simulink model "DSPequivalent_FOC_2020a"  (R2020a)
settings: Solver=ode5  StartTime=0.0  StopTime=tend  FixedStep=Tsim  RelTol=1e-3
values from neighbouring files (symbols this model uses):
  alpha = 0.091    [init_DSPeq_FOC.m]    (also in init_DSPeq_IM.m = 0.04; paramSet.m = 0.04)
  d = 0.444    [FRAexport_2.m]    (also in init_DSPeq_FOC.m = 0.78975)
  DEADTIME = 100    [init_DSPeq_FOC.m]    (also in init_DSPeq_IM.m)
  emf = psi*we    [init_DSPeq_FOC.m]
  f_ref = 270    [init_DSPeq_FOC.m]    (also in init_DSPeq_IM.m = 50)
  Id_ref = 0    [init_DSPeq_FOC.m]    (also in init_DSPeq_IM.m = 1; step_prikaz.m = Idq2(:,2))
  Iq_ref = 2    [init_DSPeq_FOC.m]    (also in init_DSPeq_IM.m = 1; step_prikaz.m = Idq2(:,3))
  ISENSE_SCALE = 10    [init_DSPeq_FOC.m]    (also in init_DSPeq_IM.m)
  Ki = 0.2/ur    (= 0.05)    [init_DSPeq.m]    (also in init_DSPeq_FOC.m = wc*Kp/(tan(-pi/2+pm+2*atan(wc*Ts/4)+atan(wc*L/R))))
  Kp = 1.8    [init_DSPeq.m]    (also in init_DSPeq_FOC.m = R*sqrt(1+(wc*L/R)^2))
  L = 3.4e-3    (= 0.0034)    [init_DSPeq_FOC.m]
  Nos = 16    [init_DSPeq.m]    (also in init_DSPeq_FOC.m; init_DSPeq_IM.m)
  ofst_a = 0    [init_DSPeq_FOC.m]
  ofst_b = 0    [init_DSPeq_FOC.m]
  OVERSAMPLING = 1    [init_DSPeq.m]    (also in init_DSPeq_FOC.m; init_DSPeq_IM.m; raw_plot.m)
  p = 3    [init_DSPeq_FOC.m]    (also in init_DSPeq_IM.m = 1)
  ph = pi    (= 3.14159265359)    [init_DSPeq_FOC.m]
  PWM_TBPRD = 4992    [init_DSPeq.m]    (also in init_DSPeq_FOC.m; init_DSPeq_IM.m; paramSet.m)
  R = 9.92e3    (= 9920)    [init_DSPeq.m]    (also in init_DSPeq_FOC.m = 0.47)
  Tadc_exe = Tadc    (= 6.24e-06)    [init_DSPeq_FOC.m]
  tau_fil = 5e-6    (= 5e-06)    [init_DSPeq_FOC.m]
  tfra = 0.33    [init_DSPeq_FOC.m]
  Tpwm = 2*PWM_TBPRD/ftbclk    (= 9.984e-05)    [init_DSPeq.m]    (also in init_DSPeq_FOC.m; init_DSPeq_IM.m; paramSet.m)
  tref = dmacnt_ref*Ts    [init_DSPeq_FOC.m]
  Ts = Tpwm/ur    (= 2.496e-05)    [init_DSPeq.m]    (also in init_DSPeq_FOC.m = 4.992e-05; init_DSPeq_IM.m = 4.992e-05; paramSet.m = 4.992e-05; step_prikaz.m = Ts/1000)
  Ts_cmp = Ts    (= 4.992e-05)    [init_DSPeq_FOC.m]
  Ts_exe = Ts    (= 4.992e-05)    [init_DSPeq_FOC.m]
  Ttbclk = 1/ftbclk    (= 1e-08)    [init_DSPeq.m]    (also in init_DSPeq_FOC.m; init_DSPeq_IM.m; paramSet.m)
  Udol = 0    [init_DSPeq_FOC.m]    (also in init_DSPeq_IM.m = UD_MAX/2)
  Udq0 = [0; 0]    [init_DSPeq_FOC.m]
  Udq_max = E/2    (= 260)    [init_DSPeq_FOC.m]    (also in init_DSPeq_IM.m = E/(2*sqrt(2)))
  Uqol = 0    [init_DSPeq_FOC.m]    (also in init_DSPeq_IM.m)
  ur = 4    [init_DSPeq.m]    (also in init_DSPeq_FOC.m = 2; init_DSPeq_IM.m = 2; paramSet.m = 2; raw_plot.m = 2)
  we = 2*pi*f_ref    (= 1696.46003294)    [init_DSPeq_FOC.m]
  wm = we/p    (= 565.486677646)    [init_DSPeq_FOC.m]
undefined symbols (not defined in the file or in its folder): j, Ld, Lq
libraries: simulink x12, powerlib x5, slctrlblks x1
settings Model: Creator=ruzic  LastModifiedBy=ruzic
settings DataIOCC: ReturnWorkspaceOutputs=off
settings DebuggingCC: UnderSpecifiedDataTypeMsg=warning  UnderSpecifiedDimensionMsg=warning  ArithmeticOperatorsInVariantConditions=warning
settings SFSimCC: CustomCodeUndefinedFunction=UseInterfaceOnly

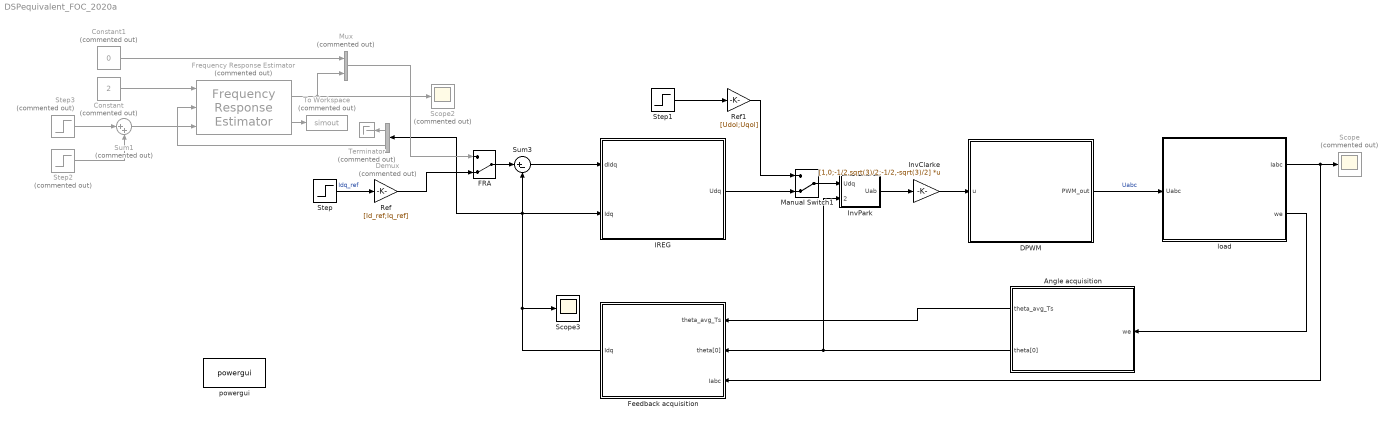
== system DSPequivalent_FOC_2020a ==
  Angle acquisition : Subsystem
  Constant : Constant  Commented=on  Value=2  SampleTime=Ts
  Constant1 : Constant  Commented=on  Value=0  SampleTime=Ts
  DPWM : Subsystem
  Demux : Demux  Commented=on  Outputs=2
  FRA : ManualSwitch  CurrentSetting=0
  Feedback acquisition : Subsystem
  Frequency Response Estimator : slctrlblks/Frequency Response Estimator  Commented=on  DiscreteTs=Ts  OutputMode=control action + perturbation  BlockDataType=double  SineSource=Block parameters  Frequencies=f_test  FreqUnits=Hz  Amplitudes=0.1  NumOfFreq=3  ExperimentMode=Sinestream  NumOfSetPeriod=2  NumOfEstPeriod=4  NumOfSlowestPeriod=3  EstimationMode=Offline  UseBodePlot=on  BaselinePlant=W1  PlotRefreshFactor=100  BodePlotChoice=VariantNull  ExperimentChoice=VariantSSNoEst  OutputChoice=VariantCandD
      settings: SourceProductBaseCode=SD
  IREG : Subsystem
  InvClarke : Gain  Gain=[1,0;-1/2,sqrt(3)/2;-1/2,-sqrt(3)/2]  Multiplication=Matrix(K*u)
  InvPark : Subsystem
  Manual Switch1 : ManualSwitch  CurrentSetting=0
  Mux : Mux  Commented=on  Inputs=2
  Ref : Gain  Gain=[Id_ref;Iq_ref]
  Ref1 : Gain  Gain=[Udol;Uqol]
  Scope : Scope  Commented=on
  Scope2 : Scope  Commented=on
  Scope3 : Scope
  Step : Step  Time=tref  Before=4/2  SampleTime=Ts_exe
  Step1 : Step  Time=Tpwm/ur  Before=Udq0  After=Udq0  SampleTime=Ts_exe
  Step2 : Step  Commented=on  Time=tref + tfra  After=-1  SampleTime=Ts
  Step3 : Step  Commented=on  Time=tref  SampleTime=Ts
  Sum1 : Sum  Commented=on  Inputs=|++
  Sum3 : Sum  Inputs=|+-
  Terminator : Terminator  Commented=on
  To Workspace : ToWorkspace  Commented=on  VariableName=simout  SaveFormat=Timeseries  SampleTime=-1
  load : Subsystem
  powergui : powerlib/powergui  Priority=1  SimulationMode=Continuous  SampleTime=50e-6  frequency=60  Iterations=50  frequencyindice=0  Pbase=100e6  ErrMax=1e-4  UnitsV=kV  UnitsW=MW  buscounter=0  FunctionMessages=off  echomessages=off  EnableUseOfTLC=off  CurrentSourceSwitches=off  DisableSnubberDevices=off  DisableRonSwitches=off  DisableVfSwitches=off  DisplayEquations=off  AutomaticDiscreteSolvers=off  SolverType=Tustin/Backward Euler (TBE)  Interpol=off  ExternalGateDelay=off  methode=off  Ts=100  x0status=blocks  SPID=on  SwTol=0  HookPort=off  NonlinearTolerance=1e-4  nMaxIteration=100  ContinueOnMaxIteration=off  RestoreLinks=warning  ResistiveCurrentMeasurement=off  Frange=[0:2:500]  Ylog=off  Xlog=on  ShowGrid=off  save=off  variable=ZData  structure=0  ZoomFFT=off  StartTime=0.0  cycles=1  DisplayStyle=1  fundamental=60  FreqAxis=off  MaxFrequency=1000  frequencyindicesteady=1  RmsSteady=1  display=off
  wires:
  Sum3/1 -> IREG/1(dIdq)
  Step/1 -> Ref/1  "Idq_ref"
  DPWM/1(PWM_out) -> load/1(Uabc)  "Uabc"
  Ref1/1 -> Manual Switch1/1
  InvPark/1(Uab) -> InvClarke/1
  InvClarke/1 -> DPWM/1(u)
  Angle acquisition/2(theta[0]) -> InvPark/2(theta), Feedback acquisition/2(theta[0])
  Step1/1 -> Ref1/1
  Feedback acquisition/1("Idq ") -> Scope3/1, IREG/2(Idq), Demux/1, Sum3/2
  Angle acquisition/1(theta_avg_Ts) -> Feedback acquisition/1(theta_avg_Ts)
  IREG/1(Udq) -> Manual Switch1/2
  Manual Switch1/1 -> InvPark/1(Udq)
  load/2(we) -> Angle acquisition/1(we)
  load/1(Iabc) -> Feedback acquisition/3(Iabc), Scope/1
  Mux/1 -> FRA/1
  Frequency Response Estimator/1 -> Mux/2, Scope2/1
  Constant/1 -> Frequency Response Estimator/1
  Demux/2 -> Frequency Response Estimator/2
  Demux/1 -> Terminator/1
  Constant1/1 -> Mux/1
  Frequency Response Estimator/2 -> To Workspace/1
  Sum1/1 -> Frequency Response Estimator/3
  Step2/1 -> Sum1/2
  Step3/1 -> Sum1/1
  FRA/1 -> Sum3/1
  Ref/1 -> FRA/2

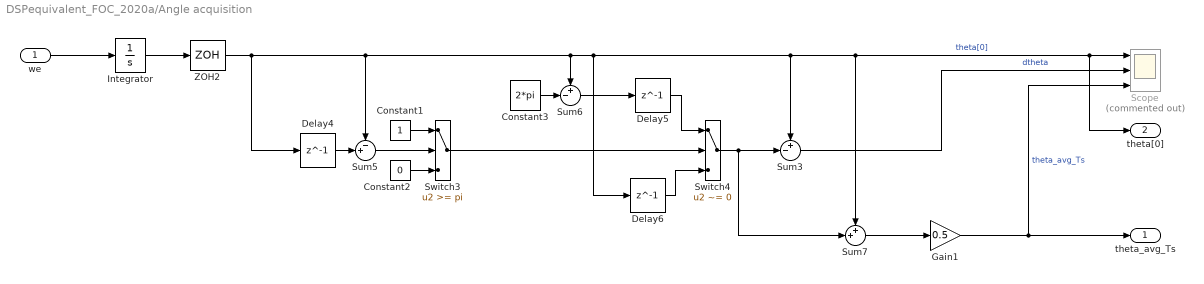
== system DSPequivalent_FOC_2020a/Angle acquisition ==
  we : Inport
  Constant1 : Constant
  Constant2 : Constant  Value=0
  Constant3 : Constant  Value=2*pi
  Delay4 : Delay  DelayLength=1
  Delay5 : Delay  DelayLength=1  SampleTime=Ts_exe
  Delay6 : Delay  DelayLength=1  SampleTime=Ts_exe
  Gain1 : Gain  Gain=0.5
  Integrator : Integrator  WrapState=on  WrappedStateUpperValue=2*pi  WrappedStateLowerValue=0
  Scope : Scope  Commented=on  NumInputPorts=3
  Sum3 : Sum  Inputs=+-|
  Sum5 : Sum  Inputs=-+|
  Sum6 : Sum  Inputs=+-|
  Sum7 : Sum  Inputs=++|
  Switch3 : Switch  Threshold=pi  OutDataTypeStr=boolean
  Switch4 : Switch  Criteria=u2 ~= 0
  ZOH2 : ZeroOrderHold  SampleTime=Ts_exe
  theta_avg_Ts : Outport  VectorParamsAs1DForOutWhenUnconnected=off
  theta[0] : Outport  Port=2  VectorParamsAs1DForOutWhenUnconnected=off
  wires:
  Integrator/1 -> ZOH2/1
  Sum3/1 -> Scope/2  "dtheta"
  Delay4/1 -> Sum5/2
  Sum5/1 -> Switch3/2
  Constant1/1 -> Switch3/1
  Constant2/1 -> Switch3/3
  Constant3/1 -> Sum6/2
  Switch3/1 -> Switch4/2
  Delay5/1 -> Switch4/1
  Switch4/1 -> Sum7/2, Sum3/2
  Delay6/1 -> Switch4/3
  Sum7/1 -> Gain1/1
  Sum6/1 -> Delay5/1
  we/1 -> Integrator/1
  ZOH2/1 -> Delay6/1, theta[0]/1, Scope/1, Sum7/1, Sum3/1, Sum6/1, Sum5/1, Delay4/1  "theta[0]"
  Gain1/1 -> theta_avg_Ts/1, Scope/3  "theta_avg_Ts"

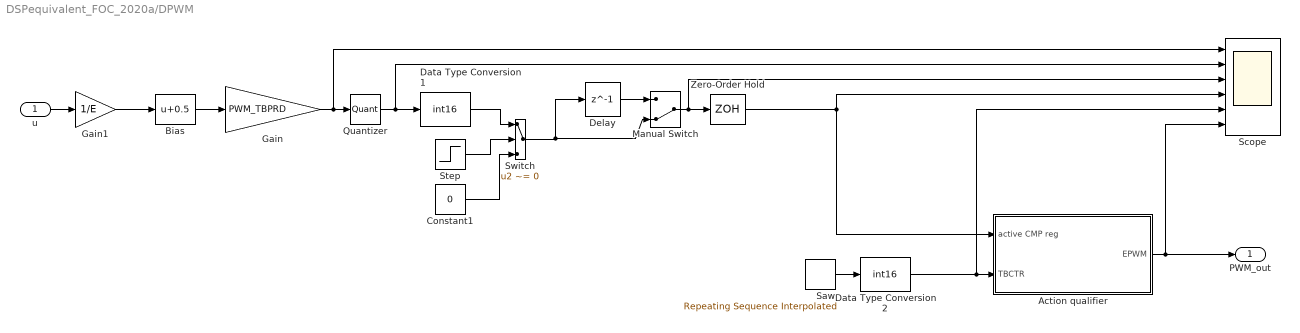
== system DSPequivalent_FOC_2020a/DPWM ==
  u : Inport
  Action qualifier : Subsystem
  Bias : Bias  Bias=0.5
  Constant1 : Constant  Value=0
  Data Type Conversion1 : DataTypeConversion  OutDataTypeStr=int16  ConvertRealWorld=Stored Integer (SI)  RndMeth=Round
  Data Type Conversion2 : DataTypeConversion  OutDataTypeStr=int16  ConvertRealWorld=Stored Integer (SI)  RndMeth=Round
  Delay : Delay  DelayLength=1  InitialCondition=0  SampleTime=Ts_exe
  Gain : Gain  Gain=PWM_TBPRD
  Gain1 : Gain  Gain=1/E
  Manual Switch : ManualSwitch  CurrentSetting=0
  Quantizer : Quantizer  QuantizationInterval=1
  Saw : simulink/Sources/Repeating Sequence Interpolated  OutValues=[0 PWM_TBPRD 1].'  TimeValues=[0 Tpwm/2 (Tpwm-Ttbclk)].'  LookUpMeth=Interpolation-Use End Values  tsamp=Ttbclk  OutMin=[]  OutMax=[]  OutDataTypeStr=double  OutputDataTypeScalingMode=double  OutDataType=fixdt(0,8)  OutScaling=2^-10
  Scope : Scope  NumInputPorts=6
  Step : Step  Time=Tpwm/ur
  Switch : Switch  Criteria=u2 ~= 0
  Zero-Order Hold : ZeroOrderHold  SampleTime=Ts_cmp
  PWM_out : Outport  VectorParamsAs1DForOutWhenUnconnected=off
  wires:
  u/1 -> Gain1/1
  Quantizer/1 -> Data Type Conversion1/1, Scope/2
  Saw/1 -> Data Type Conversion2/1
  Zero-Order Hold/1 -> Action qualifier/1(active CMP reg), Scope/4
  Action qualifier/1(EPWM) -> Scope/6, PWM_out/1
  Data Type Conversion1/1 -> Switch/1
  Data Type Conversion2/1 -> Scope/5, Action qualifier/2(TBCTR)
  Gain1/1 -> Bias/1
  Gain/1 -> Quantizer/1, Scope/1
  Bias/1 -> Gain/1
  Constant1/1 -> Switch/3
  Step/1 -> Switch/2
  Switch/1 -> Manual Switch/2, Delay/1
  Manual Switch/1 -> Scope/3, Zero-Order Hold/1
  Delay/1 -> Manual Switch/1

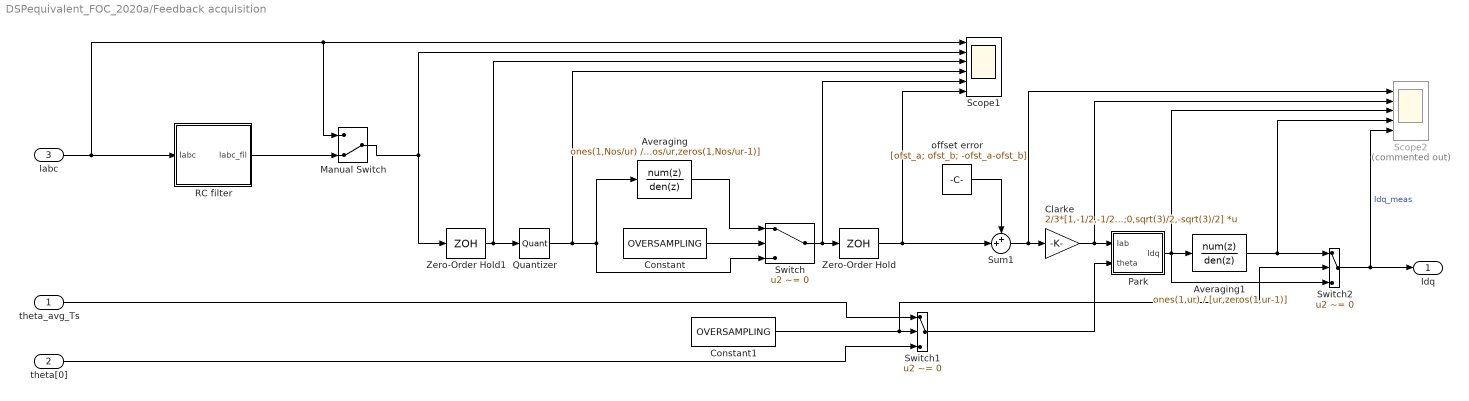
== system DSPequivalent_FOC_2020a/Feedback acquisition ==
  theta_avg_Ts : Inport
  theta[0] : Inport  Port=2
  Iabc : Inport  Port=3
  Averaging : DiscreteTransferFcn  Numerator=ones(1,Nos/ur)  Denominator=[Nos/ur,zeros(1,Nos/ur-1)]
  Averaging1 : DiscreteTransferFcn  Numerator=ones(1,ur)  Denominator=[ur,zeros(1,ur-1)]
  Clarke : Gain  Gain=2/3*[1,-1/2,-1/2;0,sqrt(3)/2,-sqrt(3)/2]  Multiplication=Matrix(K*u)
  Constant : Constant  Value=OVERSAMPLING
  Constant1 : Constant  Value=OVERSAMPLING
  Manual Switch : ManualSwitch  CurrentSetting=0
  Park : Subsystem
  Quantizer : Quantizer  QuantizationInterval=3/(2^12-1)*ISENSE_SCALE
  RC filter : Subsystem
  Scope1 : Scope  NumInputPorts=6
  Scope2 : Scope  Commented=on  NumInputPorts=5
  Sum1 : Sum  Inputs=++|
  Switch : Switch  Criteria=u2 ~= 0
  Switch1 : Switch  Criteria=u2 ~= 0
  Switch2 : Switch  Criteria=u2 ~= 0
  Zero-Order Hold : ZeroOrderHold  SampleTime=Ts_exe
  Zero-Order Hold1 : ZeroOrderHold  SampleTime=Tadc_exe
  offset error : Constant  Value=[ofst_a; ofst_b; -ofst_a-ofst_b]  SampleTime=Ts_exe
  "Idq " : Outport  VectorParamsAs1DForOutWhenUnconnected=off
  wires:
  Switch/1 -> Scope1/5, Zero-Order Hold/1
  Zero-Order Hold1/1 -> Scope1/3, Quantizer/1
  Quantizer/1 -> Scope1/4, Switch/3, Averaging/1
  Averaging/1 -> Switch/1
  Constant/1 -> Switch/2
  Constant1/1 -> Switch2/2, Switch1/2
  Switch2/1 -> Scope2/5, "Idq "/1  "Idq_meas"
  theta[0]/1 -> Switch1/3
  theta_avg_Ts/1 -> Switch1/1
  Averaging1/1 -> Scope2/4, Switch2/1
  Switch1/1 -> Park/2(theta)
  Clarke/1 -> Scope2/2, Park/1(Iab)
  Park/1(Idq) -> Switch2/3, Scope2/3, Averaging1/1
  Sum1/1 -> Scope2/1, Clarke/1
  Manual Switch/1 -> Scope1/2, Zero-Order Hold1/1
  Iabc/1 -> RC filter/1(Iabc), Manual Switch/1, Scope1/1
  RC filter/1(Iabc_fil) -> Manual Switch/2
  Zero-Order Hold/1 -> Scope1/6, Sum1/2
  offset error/1 -> Sum1/1

== system DSPequivalent_FOC_2020a/IREG ==
  dIdq : Inport
  Idq : Inport  Port=2
  Dif.comp. : Subsystem
  IMC : Subsystem
  Manual Switch : ManualSwitch
  Manual Switch1 : ManualSwitch
  PI error decoupl. : Subsystem
  PI feedback decoupl. : Subsystem
  Scope : Scope
  Udq : Outport  VectorParamsAs1DForOutWhenUnconnected=off
  wires:
  Manual Switch/1 -> Scope/1, Udq/1
  dIdq/1 -> PI feedback decoupl./1(dIdq), PI error decoupl./1(dIdq), IMC/1(dIdq)
  IMC/1(Out) -> Dif.comp./1(In)
  Dif.comp./1(Out) -> Manual Switch/1
  Idq/1 -> PI feedback decoupl./2(Idq)
  PI error decoupl./1(Out) -> Manual Switch1/1
  PI feedback decoupl./1(Out) -> Manual Switch1/2
  Manual Switch1/1 -> Manual Switch/2

== system DSPequivalent_FOC_2020a/InvPark ==
  Udq : Inport
  theta : Inport  Port=2
  Complex to Real-Imag1 : ComplexToRealImag
  Demux : Demux  Outputs=2
  Gain8 : Gain  Gain=1j
  Math Function1 : Math  SignedPower=on  OutputSignalType=complex  SaturateOnIntegerOverflow=on
  Mux3 : Mux  Inputs=2
  Product4 : Product
  Real-Imag to Complex1 : RealImagToComplex
  Uab : Outport  VectorParamsAs1DForOutWhenUnconnected=off
  wires:
  Real-Imag to Complex1/1 -> Product4/2
  Math Function1/1 -> Product4/1
  Complex to Real-Imag1/1 -> Mux3/1
  Gain8/1 -> Math Function1/1
  Demux/1 -> Real-Imag to Complex1/1  "ud"
  Mux3/1 -> Uab/1  "Uab"
  Product4/1 -> Complex to Real-Imag1/1
  Complex to Real-Imag1/2 -> Mux3/2
  Demux/2 -> Real-Imag to Complex1/2  "uq"
  theta/1 -> Gain8/1
  Udq/1 -> Demux/1

== system DSPequivalent_FOC_2020a/load ==
  Uabc : Inport
  Demux : Demux  Outputs=2
  Manual Switch : ManualSwitch  CurrentSetting=0
  Mux : Mux  Commented=on  Inputs=2
  Mux1 : Mux  Inputs=2
  PMSM : Subsystem
  RL + emf : Subsystem  Commented=on
  Iabc : Outport  VectorParamsAs1DForOutWhenUnconnected=off
  we : Outport  Port=2  VectorParamsAs1DForOutWhenUnconnected=off
  tag scope: iabc=global
  wires:
  Uabc/1 -> PMSM/1(Uabc), RL + emf/1(Uabc)
  Demux/1 -> [iabc], Iabc/1
  Mux/1 -> Manual Switch/1
  RL + emf/1(Iabc) -> Mux/1
  RL + emf/2(we) -> Mux/2
  Manual Switch/1 -> Demux/1
  Demux/2 -> we/1
  PMSM/1(Iabc) -> Mux1/1
  PMSM/2(we) -> Mux1/2
  Mux1/1 -> Manual Switch/2

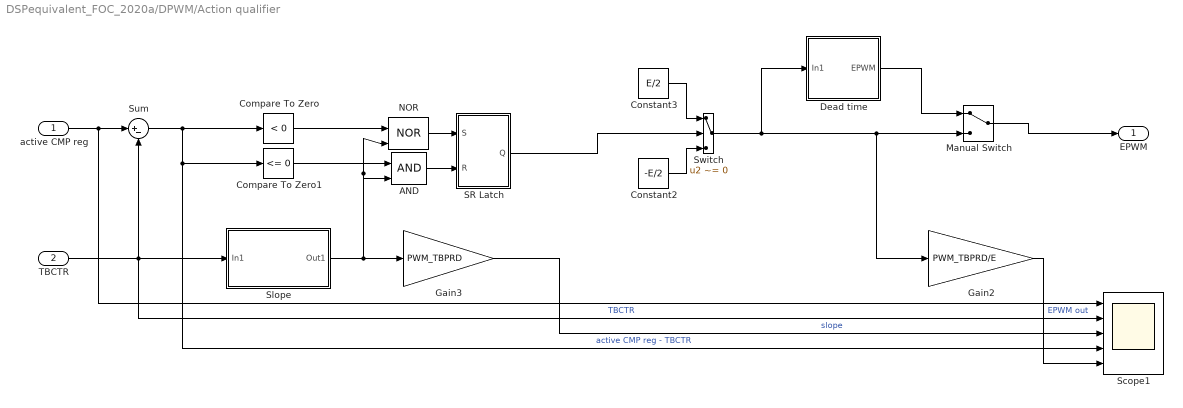
== system DSPequivalent_FOC_2020a/DPWM/Action qualifier ==
  active CMP reg : Inport
  TBCTR : Inport  Port=2
  AND : Logic  IconShape=distinctive  AllPortsSameDT=off  OutDataTypeStr=boolean
  Compare To Zero : simulink/Logic and Bit Operations/Compare To Zero  relop=<  OutDataTypeStr=boolean
  Compare To Zero1 : simulink/Logic and Bit Operations/Compare To Zero  relop=<=  OutDataTypeStr=boolean
  Constant2 : Constant  Value=-E/2
  Constant3 : Constant  Value=E/2
  Dead time : Subsystem
  Gain2 : Gain  Gain=PWM_TBPRD/E
  Gain3 : Gain  Gain=PWM_TBPRD
  Manual Switch : ManualSwitch
  NOR : Logic  Operator=NOR  IconShape=distinctive  AllPortsSameDT=off  OutDataTypeStr=boolean
  SR Latch : Subsystem
  Scope1 : Scope  NumInputPorts=5
  Slope : Subsystem
  Sum : Sum  Inputs=|+-
  Switch : Switch  Criteria=u2 ~= 0
  EPWM : Outport  VectorParamsAs1DForOutWhenUnconnected=off
  wires:
  Gain3/1 -> Scope1/3  "slope"
  active CMP reg/1 -> Scope1/1, Sum/1
  Gain2/1 -> Scope1/5  "EPWM out"
  Sum/1 -> Scope1/4, Compare To Zero1/1, Compare To Zero/1  "active CMP reg - TBCTR"
  TBCTR/1 -> Scope1/2, Slope/1(In1), Sum/2  "TBCTR"
  AND/1 -> SR Latch/2(R)
  Compare To Zero/1 -> NOR/1
  NOR/1 -> SR Latch/1(S)
  Compare To Zero1/1 -> AND/1
  Slope/1(Out1) -> Gain3/1, AND/2, NOR/2
  SR Latch/1(Q) -> Switch/2
  Constant2/1 -> Switch/3
  Constant3/1 -> Switch/1
  Manual Switch/1 -> EPWM/1
  Dead time/1(EPWM) -> Manual Switch/1
  Switch/1 -> Manual Switch/2, Gain2/1, Dead time/1(In1)

== system DSPequivalent_FOC_2020a/Feedback acquisition/Park ==
  Iab : Inport
  theta : Inport  Port=2
  Complex to Real-Imag1 : ComplexToRealImag
  Demux : Demux  Outputs=2
  Gain8 : Gain  Gain=-1j
  Math Function1 : Math  SignedPower=on  OutputSignalType=complex  SaturateOnIntegerOverflow=on
  Mux3 : Mux  Inputs=2
  Product4 : Product
  Real-Imag to Complex1 : RealImagToComplex
  Idq : Outport  VectorParamsAs1DForOutWhenUnconnected=off
  wires:
  Real-Imag to Complex1/1 -> Product4/2
  Math Function1/1 -> Product4/1
  Complex to Real-Imag1/1 -> Mux3/1
  Gain8/1 -> Math Function1/1
  theta/1 -> Gain8/1
  Demux/1 -> Real-Imag to Complex1/1  "ialfa"
  Mux3/1 -> Idq/1  "Idq"
  Product4/1 -> Complex to Real-Imag1/1
  Complex to Real-Imag1/2 -> Mux3/2
  Demux/2 -> Real-Imag to Complex1/2  "ibeta"
  Iab/1 -> Demux/1

== system DSPequivalent_FOC_2020a/Feedback acquisition/RC filter ==
  Iabc : Inport
  Demux : Demux  Outputs=3
  Mux : Mux  Inputs=3
  Transfer Fcn1 : TransferFcn  Denominator=[tau_fil 1]
  Transfer Fcn2 : TransferFcn  Denominator=[tau_fil 1]
  Transfer Fcn3 : TransferFcn  Denominator=[tau_fil 1]
  Iabc_fil : Outport  VectorParamsAs1DForOutWhenUnconnected=off
  wires:
  Transfer Fcn3/1 -> Mux/1
  Mux/1 -> Iabc_fil/1
  Demux/3 -> Transfer Fcn2/1
  Transfer Fcn1/1 -> Mux/2
  Iabc/1 -> Demux/1
  Demux/1 -> Transfer Fcn3/1
  Transfer Fcn2/1 -> Mux/3
  Demux/2 -> Transfer Fcn1/1

== system DSPequivalent_FOC_2020a/IREG/Dif.comp. ==
  In : Inport
  Difference : simulink/Discrete/Difference  ICPrevInput=0.0  OutMin=[]  OutMax=[]  OutDataType=fixdt(1, 16)  OutScaling=2^-10  DoSatur=off
  Gain : Gain  Gain=d
  Sum1 : Sum  Inputs=|++
  Out : Outport
  wires:
  Gain/1 -> Sum1/1
  In/1 -> Sum1/2, Difference/1
  Difference/1 -> Gain/1
  Sum1/1 -> Out/1

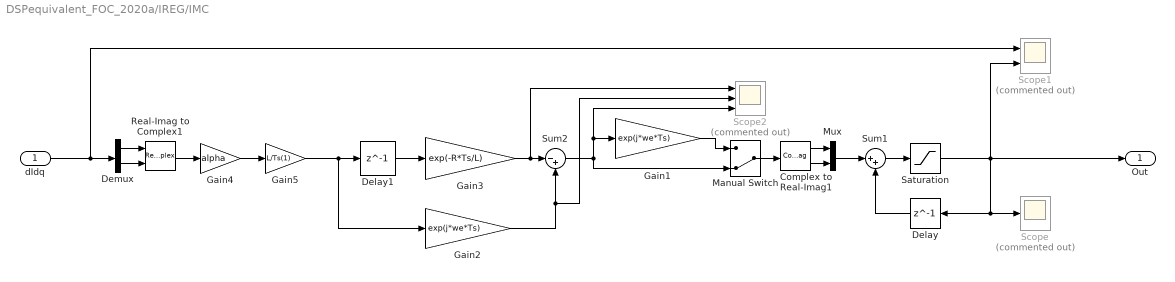
== system DSPequivalent_FOC_2020a/IREG/IMC ==
  dIdq : Inport
  Complex to Real-Imag1 : ComplexToRealImag
  Delay : Delay  DelayLength=1  InitialCondition=Udq0
  Delay1 : Delay  DelayLength=1
  Demux : Demux  Outputs=2
  Gain1 : Gain  Gain=exp(j*we*Ts)
  Gain2 : Gain  Gain=exp(j*we*Ts)
  Gain3 : Gain  Gain=exp(-R*Ts/L)
  Gain4 : Gain  Gain=alpha
  Gain5 : Gain  Gain=L/Ts(1)
  Manual Switch : ManualSwitch  CurrentSetting=0
  Mux : Mux  Inputs=2
  Real-Imag to Complex1 : RealImagToComplex
  Saturation : Saturate  UpperLimit=Udq_max  LowerLimit=-Udq_max
  Scope : Scope  Commented=on
  Scope1 : Scope  Commented=on  NumInputPorts=2
  Scope2 : Scope  Commented=on  NumInputPorts=3
  Sum1 : Sum  Inputs=|++
  Sum2 : Sum  Inputs=|-+
  Out : Outport
  wires:
  Gain2/1 -> Sum2/2, Scope2/2
  Delay/1 -> Sum1/2
  Demux/1 -> Real-Imag to Complex1/1
  Gain5/1 -> Gain2/1, Delay1/1
  Sum2/1 -> Manual Switch/2, Scope2/3, Gain1/1
  dIdq/1 -> Demux/1, Scope1/1
  Demux/2 -> Real-Imag to Complex1/2
  Delay1/1 -> Gain3/1
  Mux/1 -> Sum1/1
  Saturation/1 -> Out/1, Scope1/2, Delay/1, Scope/1
  Complex to Real-Imag1/1 -> Mux/1
  Gain3/1 -> Scope2/1, Sum2/1
  Real-Imag to Complex1/1 -> Gain4/1
  Complex to Real-Imag1/2 -> Mux/2
  Gain4/1 -> Gain5/1
  Sum1/1 -> Saturation/1
  Gain1/1 -> Manual Switch/1
  Manual Switch/1 -> Complex to Real-Imag1/1

== system DSPequivalent_FOC_2020a/IREG/PI error decoupl. ==
  dIdq : Inport
  Manual Switch : ManualSwitch  CurrentSetting=0
  PI err KpKi classic : Subsystem
  PI err RL : Subsystem
  Out : Outport
  wires:
  dIdq/1 -> PI err RL/1(dIdq), PI err KpKi classic/1(In1)
  PI err KpKi classic/1(Out1) -> Manual Switch/1
  PI err RL/1(Out1) -> Manual Switch/2
  Manual Switch/1 -> Out/1

== system DSPequivalent_FOC_2020a/IREG/PI feedback decoupl. ==
  dIdq : Inport
  Idq : Inport  Port=2
  Manual Switch : ManualSwitch  CurrentSetting=0
  PI fb KpKi classic : Subsystem
  PI fb RL : Subsystem
  Out : Outport
  wires:
  Idq/1 -> PI fb RL/1(Idq), PI fb KpKi classic/1(Idq)
  dIdq/1 -> PI fb RL/2(dIdq), PI fb KpKi classic/2(dIdq)
  PI fb KpKi classic/1(Out1) -> Manual Switch/1
  Manual Switch/1 -> Out/1
  PI fb RL/1(Out1) -> Manual Switch/2

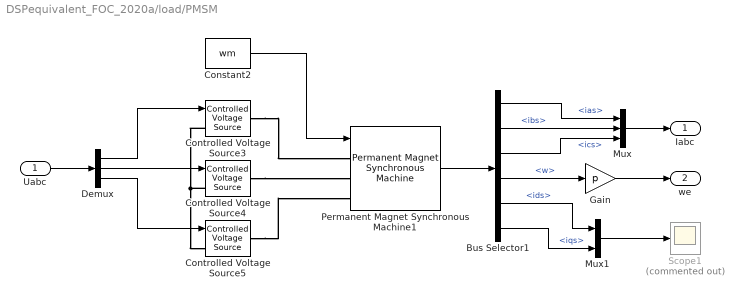
== system DSPequivalent_FOC_2020a/load/PMSM ==
  Uabc : Inport
  Bus Selector1 : BusSelector  OutputSignals=ias,ibs,ics,w,ids,iqs
  Constant2 : Constant  Value=wm
  Controlled Voltage Source3 : powerlib/Electrical Sources/Controlled Voltage Source  Initialize=on  Source_Type=AC  Amplitude=0  Phase=0  Frequency=0  Measurements=None
  Controlled Voltage Source4 : powerlib/Electrical Sources/Controlled Voltage Source  Initialize=on  Source_Type=AC  Amplitude=0  Phase=0  Frequency=0  Measurements=None
  Controlled Voltage Source5 : powerlib/Electrical Sources/Controlled Voltage Source  Initialize=on  Source_Type=AC  Amplitude=0  Phase=0  Frequency=0  Measurements=None
  Demux : Demux  Outputs=3
  Gain : Gain  Gain=p
  Mux : Mux  Inputs=3
  Mux1 : Mux  Inputs=2
  Permanent Magnet Synchronous Machine1 : powerlib/Machines/Permanent Magnet Synchronous Machine  NbPhases=3  FluxDistribution=Sinusoidal  RotorType=Round  MechanicalLoad=Speed w  PresetModel=No  ShowDetailedParameters=on  MeasurementBus=on  Resistance=R  Inductance=8.5e-3  dqInductances=[Ld,Lq]  La=L  MachineConstant=Flux linkage established by magnets (V.s)  Flux=0.1322  VoltageCst=71.9353  TorqueCst=0.5949  Flat=120  Mechanical=[0.0027 0 6 0]  PolePairs=p  InitialConditions=[wm,0, 0,0]  InitialConditions5ph=[0 0 0 0 0 0]  RefAngle=Aligned with phase A axis (original Park)  IterativeDiscreteModel=Trapezoidal non iterative  TsBlock=-1  TsPowergui=0
  Scope1 : Scope  Commented=on
  Iabc : Outport  VectorParamsAs1DForOutWhenUnconnected=off
  we : Outport  Port=2  VectorParamsAs1DForOutWhenUnconnected=off
  wires:
  Constant2/1 -> Permanent Magnet Synchronous Machine1/1
  Demux/2 -> Controlled Voltage Source4/1
  Demux/1 -> Controlled Voltage Source3/1
  Demux/3 -> Controlled Voltage Source5/1
  Uabc/1 -> Demux/1
  Permanent Magnet Synchronous Machine1/1 -> Bus Selector1/1
  Bus Selector1/2 -> Mux/2  "<ibs>"
  Mux/1 -> Iabc/1
  Bus Selector1/4 -> Gain/1  "<w>"
  Bus Selector1/1 -> Mux/1  "<ias>"
  Bus Selector1/3 -> Mux/3  "<ics>"
  Gain/1 -> we/1
  Bus Selector1/5 -> Mux1/1  "<ids>"
  Bus Selector1/6 -> Mux1/2  "<iqs>"
  Mux1/1 -> Scope1/1
  connections:
  Controlled Voltage Source4/RConn1 -- Permanent Magnet Synchronous Machine1/LConn2
  Controlled Voltage Source4/LConn1 -- Controlled Voltage Source3/LConn1 -- Controlled Voltage Source5/LConn1
  Controlled Voltage Source3/RConn1 -- Permanent Magnet Synchronous Machine1/LConn1
  Controlled Voltage Source5/RConn1 -- Permanent Magnet Synchronous Machine1/LConn3

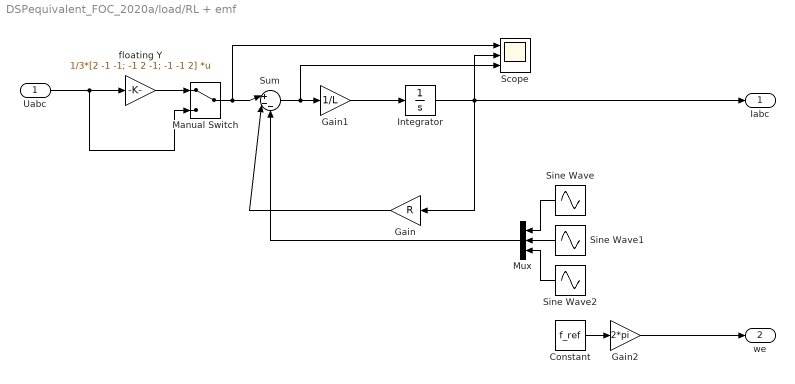
== system DSPequivalent_FOC_2020a/load/RL + emf ==
  Uabc : Inport
  Constant : Constant  Value=f_ref
  Gain : Gain  Gain=R
  Gain1 : Gain  Gain=1/L
  Gain2 : Gain  Gain=2*pi
  Integrator : Integrator
  Manual Switch : ManualSwitch
  Mux : Mux  Inputs=3
  Scope : Scope  NumInputPorts=3
  Sine Wave : Sin  Amplitude=emf  Frequency=we  Phase=ph  SampleTime=0
  Sine Wave1 : Sin  Amplitude=emf  Frequency=we  Phase=ph-2*pi/3  SampleTime=0
  Sine Wave2 : Sin  Amplitude=emf  Frequency=we  Phase=ph+2*pi/3  SampleTime=0
  Sum : Sum  Inputs=|+--
  floating Y : Gain  Gain=1/3*[2 -1 -1; -1 2 -1; -1 -1 2]  Multiplication=Matrix(K*u)
  Iabc : Outport  VectorParamsAs1DForOutWhenUnconnected=off
  we : Outport  Port=2  VectorParamsAs1DForOutWhenUnconnected=off
  wires:
  Uabc/1 -> Manual Switch/2, floating Y/1
  Gain1/1 -> Integrator/1
  Integrator/1 -> Scope/2, Gain/1, Iabc/1
  Constant/1 -> Gain2/1
  Gain/1 -> Sum/2
  Mux/1 -> Sum/3
  Gain2/1 -> we/1
  Sum/1 -> Scope/3, Gain1/1
  floating Y/1 -> Manual Switch/1
  Sine Wave/1 -> Mux/1
  Sine Wave1/1 -> Mux/2
  Sine Wave2/1 -> Mux/3
  Manual Switch/1 -> Scope/1, Sum/1

== system DSPequivalent_FOC_2020a/DPWM/Action qualifier/Dead time ==
  In1 : Inport
  Bias : Bias  Bias=0.5
  Delay1 : Delay  DelayLength=DEADTIME  SampleTime=Ttbclk
  Gain : Gain  Gain=1/E
  Gain1 : Gain  Gain=-E/2
  OR : Logic  Operator=OR  IconShape=distinctive  AllPortsSameDT=off  OutDataTypeStr=boolean
  SR Latch : Subsystem
  Scope : Scope  NumInputPorts=4
  Sign : Signum
  Switch1 : Switch  Criteria=u2 ~= 0
  neg edge det : Subsystem
  pos edge det : Subsystem
  EPWM : Outport  VectorParamsAs1DForOutWhenUnconnected=off
  wires:
  neg edge det/1(Out1) -> OR/2
  pos edge det/1(Out1) -> OR/1
  Delay1/1 -> SR Latch/2(R)
  OR/1 -> SR Latch/1(S), Delay1/1
  SR Latch/1(Q) -> Switch1/2
  Switch1/1 -> Scope/4, EPWM/1
  In1/1 -> Switch1/3, Scope/1, Gain/1
  Gain/1 -> Bias/1
  Bias/1 -> neg edge det/1(In1), pos edge det/1(In1)
  [iabc] -> Scope/2, Sign/1
  Sign/1 -> Gain1/1
  Gain1/1 -> Scope/3, Switch1/1

== system DSPequivalent_FOC_2020a/DPWM/Action qualifier/SR Latch ==
  S : Inport
  R : Inport  Port=2
  AND1 : Logic  IconShape=distinctive  AllPortsSameDT=off  OutDataTypeStr=boolean
  Memory : Memory
  NOT : Logic  Operator=NOT  IconShape=distinctive  AllPortsSameDT=off  OutDataTypeStr=boolean
  OR : Logic  Operator=OR  IconShape=distinctive  AllPortsSameDT=off  OutDataTypeStr=boolean
  Q : Outport  VectorParamsAs1DForOutWhenUnconnected=off
  wires:
  AND1/1 -> Q/1, Memory/1
  R/1 -> NOT/1
  S/1 -> OR/2
  OR/1 -> AND1/1
  NOT/1 -> AND1/2
  Memory/1 -> OR/1

== system DSPequivalent_FOC_2020a/DPWM/Action qualifier/Slope ==
  In1 : Inport
  AND : Logic  IconShape=distinctive  AllPortsSameDT=off  OutDataTypeStr=boolean
  Compare To Constant : simulink/Logic and Bit Operations/Compare To Constant  relop===  const=PWM_TBPRD  OutDataTypeStr=boolean
  Compare To Zero : simulink/Logic and Bit Operations/Compare To Zero  relop=~=  OutDataTypeStr=boolean
  Compare To Zero1 : simulink/Logic and Bit Operations/Compare To Zero  relop=<  OutDataTypeStr=boolean
  Difference : simulink/Discrete/Difference  ICPrevInput=0  OutMin=[]  OutMax=[]  OutDataTypeStr=int16  OutputDataTypeScalingMode=int16  OutDataType=fixdt(1, 16)  OutScaling=2^-10  DoSatur=off
  NOT : Logic  Operator=NOT  IconShape=distinctive  AllPortsSameDT=off  OutDataTypeStr=boolean
  OR : Logic  Operator=OR  IconShape=distinctive  AllPortsSameDT=off  OutDataTypeStr=boolean
  Out1 : Outport  VectorParamsAs1DForOutWhenUnconnected=off
  wires:
  In1/1 -> Difference/1, Compare To Constant/1, Compare To Zero/1
  AND/1 -> OR/1
  Compare To Zero1/1 -> AND/1
  Compare To Constant/1 -> OR/2
  Difference/1 -> Compare To Zero1/1
  OR/1 -> NOT/1
  Compare To Zero/1 -> AND/2
  NOT/1 -> Out1/1

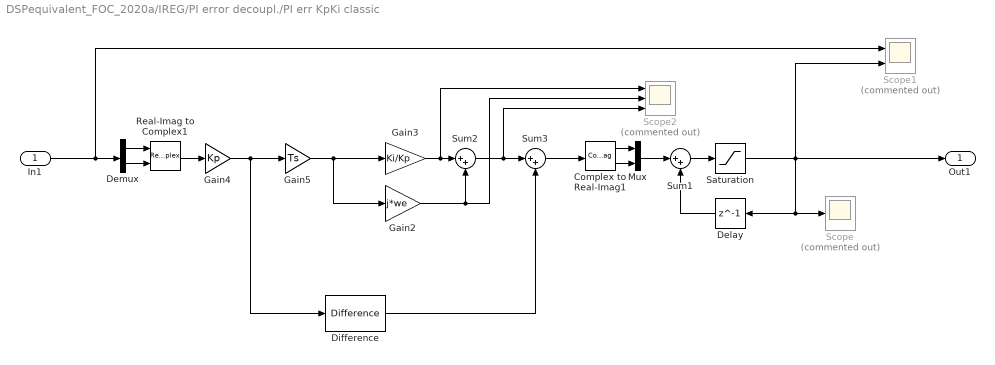
== system DSPequivalent_FOC_2020a/IREG/PI error decoupl./PI err KpKi classic ==
  In1 : Inport
  Complex to Real-Imag1 : ComplexToRealImag
  Delay : Delay  DelayLength=1  InitialCondition=Udq0
  Demux : Demux  Outputs=2
  Difference : simulink/Discrete/Difference  ICPrevInput=0.0  OutMin=[]  OutMax=[]  OutDataType=fixdt(1, 16)  OutScaling=2^-10  DoSatur=off
  Gain2 : Gain  Gain=j*we
  Gain3 : Gain  Gain=Ki/Kp
  Gain4 : Gain  Gain=Kp
  Gain5 : Gain  Gain=Ts
  Mux : Mux  Inputs=2
  Real-Imag to Complex1 : RealImagToComplex
  Saturation : Saturate  UpperLimit=Udq_max  LowerLimit=-Udq_max
  Scope : Scope  Commented=on
  Scope1 : Scope  Commented=on  NumInputPorts=2
  Scope2 : Scope  Commented=on  NumInputPorts=3
  Sum1 : Sum  Inputs=|++
  Sum2 : Sum  Inputs=|++
  Sum3 : Sum  Inputs=|++
  Out1 : Outport
  wires:
  Difference/1 -> Sum3/2
  Saturation/1 -> Out1/1, Scope1/2, Delay/1, Scope/1
  Demux/2 -> Real-Imag to Complex1/2
  Gain5/1 -> Gain2/1, Gain3/1
  Delay/1 -> Sum1/2
  Real-Imag to Complex1/1 -> Gain4/1
  Sum3/1 -> Complex to Real-Imag1/1
  Sum2/1 -> Sum3/1, Scope2/3
  Mux/1 -> Sum1/1
  Gain4/1 -> Difference/1, Gain5/1
  Demux/1 -> Real-Imag to Complex1/1
  Gain3/1 -> Scope2/1, Sum2/1
  In1/1 -> Demux/1, Scope1/1
  Gain2/1 -> Sum2/2, Scope2/2
  Complex to Real-Imag1/1 -> Mux/1
  Complex to Real-Imag1/2 -> Mux/2
  Sum1/1 -> Saturation/1

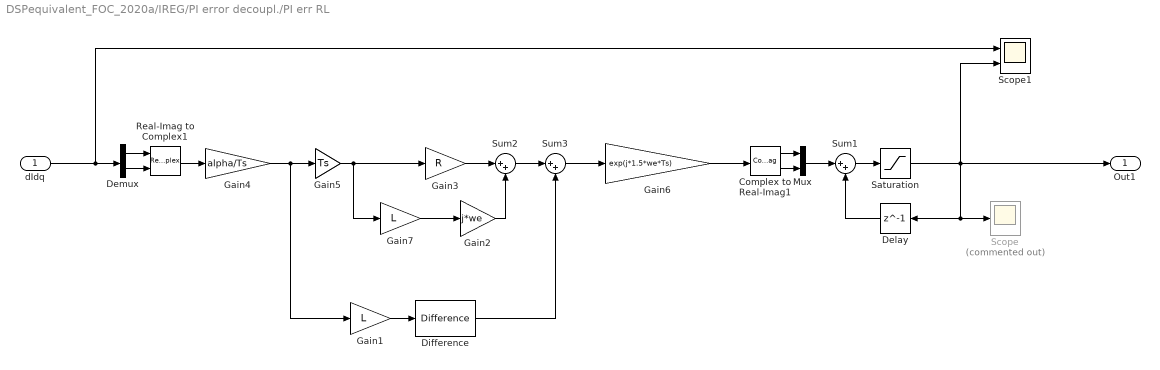
== system DSPequivalent_FOC_2020a/IREG/PI error decoupl./PI err RL ==
  dIdq : Inport
  Complex to Real-Imag1 : ComplexToRealImag
  Delay : Delay  DelayLength=1  InitialCondition=Udq0
  Demux : Demux  Outputs=2
  Difference : simulink/Discrete/Difference  ICPrevInput=0.0  OutMin=[]  OutMax=[]  OutDataType=fixdt(1, 16)  OutScaling=2^-10  DoSatur=off
  Gain1 : Gain  Gain=L
  Gain2 : Gain  Gain=j*we
  Gain3 : Gain  Gain=R
  Gain4 : Gain  Gain=alpha/Ts
  Gain5 : Gain  Gain=Ts
  Gain6 : Gain  Gain=exp(j*1.5*we*Ts)
  Gain7 : Gain  Gain=L
  Mux : Mux  Inputs=2
  Real-Imag to Complex1 : RealImagToComplex
  Saturation : Saturate  UpperLimit=Udq_max  LowerLimit=-Udq_max
  Scope : Scope  Commented=on
  Scope1 : Scope  NumInputPorts=2
  Sum1 : Sum  Inputs=|++
  Sum2 : Sum  Inputs=|++
  Sum3 : Sum  Inputs=|++
  Out1 : Outport
  wires:
  Difference/1 -> Sum3/2
  Saturation/1 -> Out1/1, Scope1/2, Delay/1, Scope/1
  Demux/2 -> Real-Imag to Complex1/2
  Gain5/1 -> Gain3/1, Gain7/1
  Delay/1 -> Sum1/2
  Real-Imag to Complex1/1 -> Gain4/1
  Sum3/1 -> Gain6/1
  Sum2/1 -> Sum3/1
  Mux/1 -> Sum1/1
  Gain4/1 -> Gain1/1, Gain5/1
  Demux/1 -> Real-Imag to Complex1/1
  Gain3/1 -> Sum2/1
  dIdq/1 -> Demux/1, Scope1/1
  Gain2/1 -> Sum2/2
  Complex to Real-Imag1/1 -> Mux/1
  Complex to Real-Imag1/2 -> Mux/2
  Sum1/1 -> Saturation/1
  Gain1/1 -> Difference/1
  Gain6/1 -> Complex to Real-Imag1/1
  Gain7/1 -> Gain2/1

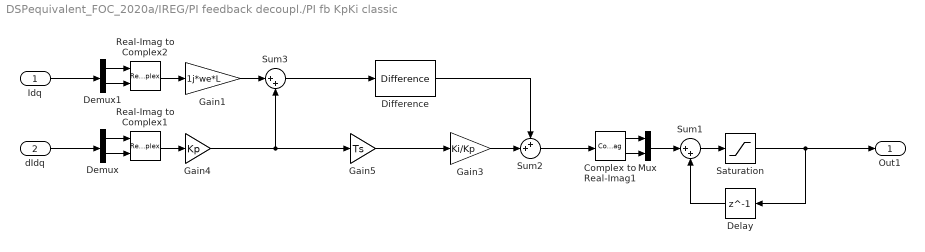
== system DSPequivalent_FOC_2020a/IREG/PI feedback decoupl./PI fb KpKi classic ==
  Idq : Inport
  dIdq : Inport  Port=2
  Complex to Real-Imag1 : ComplexToRealImag
  Delay : Delay  DelayLength=1  InitialCondition=Udq0
  Demux : Demux  Outputs=2
  Demux1 : Demux  Outputs=2
  Difference : simulink/Discrete/Difference  ICPrevInput=0.0  OutMin=[]  OutMax=[]  OutDataType=fixdt(1, 16)  OutScaling=2^-10  DoSatur=off
  Gain1 : Gain  Gain=1j*we*L
  Gain3 : Gain  Gain=Ki/Kp
  Gain4 : Gain  Gain=Kp
  Gain5 : Gain  Gain=Ts
  Mux : Mux  Inputs=2
  Real-Imag to Complex1 : RealImagToComplex
  Real-Imag to Complex2 : RealImagToComplex
  Saturation : Saturate  UpperLimit=Udq_max  LowerLimit=-Udq_max
  Sum1 : Sum  Inputs=|++
  Sum2 : Sum  Inputs=++|
  Sum3 : Sum  Inputs=|++
  Out1 : Outport
  wires:
  Demux/2 -> Real-Imag to Complex1/2
  Delay/1 -> Sum1/2
  Demux1/1 -> Real-Imag to Complex2/1
  Demux/1 -> Real-Imag to Complex1/1
  Complex to Real-Imag1/1 -> Mux/1
  Sum2/1 -> Complex to Real-Imag1/1
  Sum3/1 -> Difference/1
  Mux/1 -> Sum1/1
  Saturation/1 -> Out1/1, Delay/1
  Complex to Real-Imag1/2 -> Mux/2
  Real-Imag to Complex1/1 -> Gain4/1
  Sum1/1 -> Saturation/1
  Demux1/2 -> Real-Imag to Complex2/2
  Difference/1 -> Sum2/1
  Gain3/1 -> Sum2/2
  Gain4/1 -> Sum3/2, Gain5/1
  Idq/1 -> Demux1/1
  Real-Imag to Complex2/1 -> Gain1/1
  Gain5/1 -> Gain3/1
  Gain1/1 -> Sum3/1
  dIdq/1 -> Demux/1

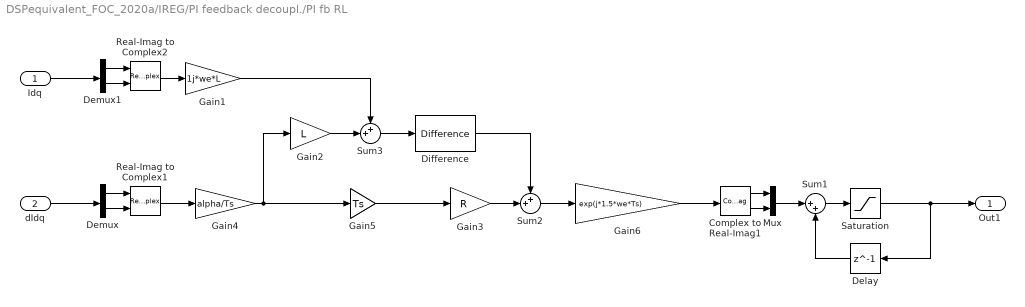
== system DSPequivalent_FOC_2020a/IREG/PI feedback decoupl./PI fb RL ==
  Idq : Inport
  dIdq : Inport  Port=2
  Complex to Real-Imag1 : ComplexToRealImag
  Delay : Delay  DelayLength=1  InitialCondition=Udq0
  Demux : Demux  Outputs=2
  Demux1 : Demux  Outputs=2
  Difference : simulink/Discrete/Difference  ICPrevInput=0.0  OutMin=[]  OutMax=[]  OutDataType=fixdt(1, 16)  OutScaling=2^-10  DoSatur=off
  Gain1 : Gain  Gain=1j*we*L
  Gain2 : Gain  Gain=L
  Gain3 : Gain  Gain=R
  Gain4 : Gain  Gain=alpha/Ts
  Gain5 : Gain  Gain=Ts
  Gain6 : Gain  Gain=exp(j*1.5*we*Ts)
  Mux : Mux  Inputs=2
  Real-Imag to Complex1 : RealImagToComplex
  Real-Imag to Complex2 : RealImagToComplex
  Saturation : Saturate  UpperLimit=Udq_max  LowerLimit=-Udq_max
  Sum1 : Sum  Inputs=|++
  Sum2 : Sum  Inputs=++|
  Sum3 : Sum  Inputs=++|
  Out1 : Outport
  wires:
  Demux/2 -> Real-Imag to Complex1/2
  Delay/1 -> Sum1/2
  Demux/1 -> Real-Imag to Complex1/1
  Complex to Real-Imag1/1 -> Mux/1
  Sum2/1 -> Gain6/1
  Gain4/1 -> Gain2/1, Gain5/1
  Mux/1 -> Sum1/1
  Saturation/1 -> Out1/1, Delay/1
  Complex to Real-Imag1/2 -> Mux/2
  Real-Imag to Complex1/1 -> Gain4/1
  Sum1/1 -> Saturation/1
  Difference/1 -> Sum2/1
  Gain3/1 -> Sum2/2
  Gain5/1 -> Gain3/1
  dIdq/1 -> Demux/1
  Sum3/1 -> Difference/1
  Gain6/1 -> Complex to Real-Imag1/1
  Gain2/1 -> Sum3/2
  Idq/1 -> Demux1/1
  Real-Imag to Complex2/1 -> Gain1/1
  Demux1/1 -> Real-Imag to Complex2/1
  Demux1/2 -> Real-Imag to Complex2/2
  Gain1/1 -> Sum3/1

== system DSPequivalent_FOC_2020a/DPWM/Action qualifier/Dead time/SR Latch ==
  S : Inport
  R : Inport  Port=2
  AND1 : Logic  IconShape=distinctive  AllPortsSameDT=off  OutDataTypeStr=boolean
  Memory : Memory
  NOT : Logic  Operator=NOT  IconShape=distinctive  AllPortsSameDT=off  OutDataTypeStr=boolean
  OR : Logic  Operator=OR  IconShape=distinctive  AllPortsSameDT=off  OutDataTypeStr=boolean
  Q : Outport  VectorParamsAs1DForOutWhenUnconnected=off
  wires:
  AND1/1 -> Q/1, Memory/1
  R/1 -> NOT/1
  S/1 -> OR/2
  OR/1 -> AND1/1
  NOT/1 -> AND1/2
  Memory/1 -> OR/1

== system DSPequivalent_FOC_2020a/DPWM/Action qualifier/Dead time/neg edge det ==
  In1 : Inport
  AND : Logic  IconShape=distinctive  AllPortsSameDT=off  OutDataTypeStr=boolean
  Memory : Memory
  NOT : Logic  Operator=NOT  IconShape=distinctive  AllPortsSameDT=off  OutDataTypeStr=boolean
  Out1 : Outport  VectorParamsAs1DForOutWhenUnconnected=off
  wires:
  Memory/1 -> AND/1
  In1/1 -> NOT/1, Memory/1
  AND/1 -> Out1/1
  NOT/1 -> AND/2

== system DSPequivalent_FOC_2020a/DPWM/Action qualifier/Dead time/pos edge det ==
  In1 : Inport
  AND : Logic  IconShape=distinctive  AllPortsSameDT=off  OutDataTypeStr=boolean
  Memory : Memory
  NOT : Logic  Operator=NOT  IconShape=distinctive  AllPortsSameDT=off  OutDataTypeStr=boolean
  Out1 : Outport  VectorParamsAs1DForOutWhenUnconnected=off
  wires:
  NOT/1 -> AND/1
  Memory/1 -> NOT/1
  In1/1 -> AND/2, Memory/1
  AND/1 -> Out1/1
